simulink model "cone"  (R2021a)
settings: Solver=VariableStepAuto  StartTime=0.0  StopTime=60  RelTol=1e-3
values from neighbouring files (symbols this model uses):
  V_init = 0.000832843134598    [cone.mat]
  V_max = 0.0439194621761    [cone.mat]
settings Model: Creator=dylan  LastModifiedBy=dylan

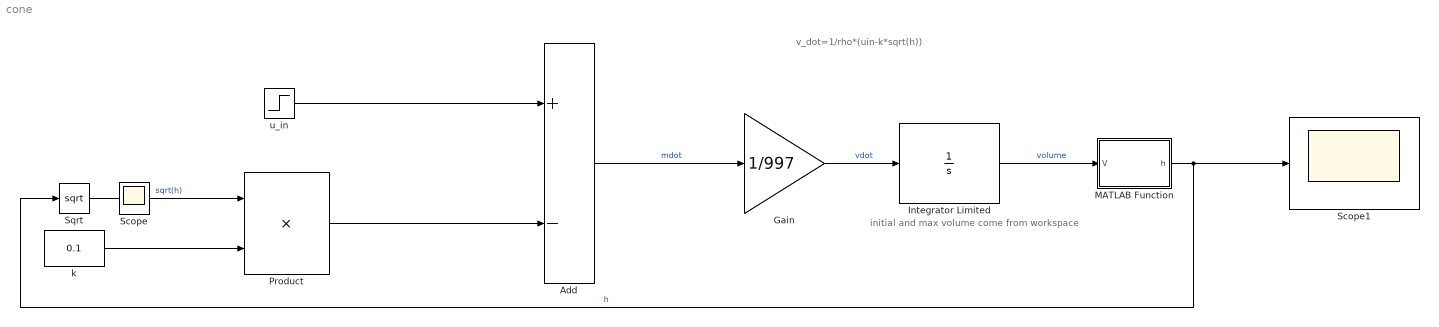
== system cone ==
  note: initial and max volume come from workspace
  note: v_dot=1/rho*(uin-k*sqrt(h))
  Add : Sum  Inputs=+-
  Gain : Gain  Gain=1/997
  Integrator Limited : Integrator  InitialCondition=V_init  LimitOutput=on  UpperSaturationLimit=V_max  LowerSaturationLimit=0
  MATLAB Function : MATLAB Function  TreatAsAtomicUnit=on
  Product : Product
  Scope : Scope
  Scope1 : Scope
  Sqrt : Sqrt  SaturateOnIntegerOverflow=on
  k : Constant  Value=0.1
  u_in : Step  Time=20  After=2  SampleTime=0
  wires:
  MATLAB Function/1(h) -> Scope1/1, Sqrt/1  "h"
  Sqrt/1 -> Product/1  "sqrt(h)"
  k/1 -> Product/2
  u_in/1 -> Add/1
  Product/1 -> Add/2
  Add/1 -> Gain/1  "mdot"
  Gain/1 -> Integrator Limited/1  "vdot"
  Integrator Limited/1 -> MATLAB Function/1(V)  "volume"

== matlab function cone/MATLAB Function ==
  data: V input; h output
function h= gethfromV(V)
h=((3*V)/(pi*(tan((7*pi)/72))^2))^(1/3);
